simulink library "alfa_window_in"  (R2013b)
settings: Solver=ode45  StartTime=0.0  StopTime=10.0  RelTol=1e-3
settings Model: Creator=lena.frank  LastModifiedBy=drhf

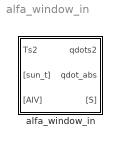
== system alfa_window_in ==
  alfa_window_in : Subsystem  mask(ALFA){gvalue=0.7, emission_in=0.87, wallsurface=1, frame=0.1, numlayer=2}
      mask prompts: gvalue "Energy transmission by sunlight (g-value) 0..1"; emission_in "Longwave emissivity (0..1)"; wallsurface "Surface of the window (with frame) in m²"; frame "Share of the frame on the surface (0...1)"; numlayer "Number of glass panes"
      mask help:
      | Convective and radiative heat transfer at the INDOOR SURFACE OF A VERTICAL WINDOW with 1-4 layers (each 3 ... 8 mm thick).
      |
      | Ts  : temperature of window surface, °C,
      | [sun_t]  : sun data (incidence angle, direct and diffuse radiation
      |     at tilted window surface),
      | [AIV]  : conditions of zone node,
      | qdots  : specific heat flow into window construction, W/m^2,
      | qdot_abs : specific irradiation absorption within window
      |     construction,  W/m^2,
      | [S]  : heat and air flow to zone node.

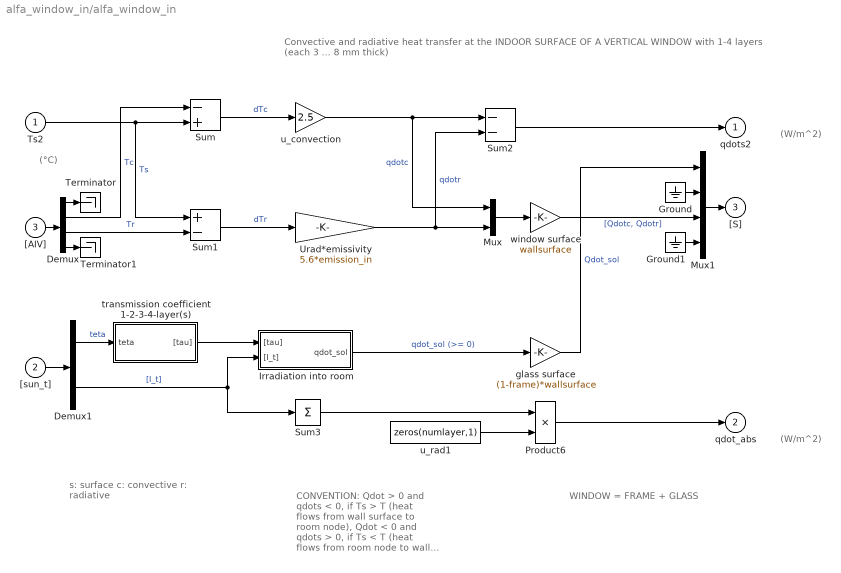
== system alfa_window_in/alfa_window_in ==
  note: (°C)
  note: Convective and radiative heat transfer at the INDOOR SURFACE OF A VERTICAL WINDOW
      | with 1-4 layers (each 3 ... 8 mm thick)
  note: (W/m^2)
  note: WINDOW = FRAME + GLASS
  note: s: surface
      | c: convective
      | r: radiative
  note: CONVENTION:
      | Qdot > 0 and qdots < 0, if Ts > T (heat flows from wall surface to room node),
      | Qdot < 0 and qdots > 0, if Ts < T (heat flows from room node to wall surface).
  note: (W/m^2)
  Ts2 : Inport
  "[sun_t]" : Inport  Port=2
  "[AIV]" : Inport  Port=3
  " glass surface" : Gain  Gain=(1-frame)*wallsurface  SaturateOnIntegerOverflow=on  OutDataTypeStr=Inherit: Same as input  ParamDataTypeStr=Inherit: Same as input
  Demux : Demux  Outputs=[1 1 1 6]
  Demux1 : Demux  Outputs=[1 2]
  Ground : Ground
  Ground1 : Ground
  Irradiation into room : Subsystem
  Mux : Mux  Inputs=2
  Mux1 : Mux  Inputs=[1 5 2 5]
  Product6 : Product  SaturateOnIntegerOverflow=on  InputSameDT=on  OutDataTypeStr=Inherit: Same as first input
  Sum : Sum  Inputs=-+  SaturateOnIntegerOverflow=on  InputSameDT=on  OutDataTypeStr=Inherit: Same as first input
  Sum1 : Sum  Inputs=+-  SaturateOnIntegerOverflow=on  InputSameDT=on  OutDataTypeStr=Inherit: Same as first input
  Sum2 : Sum  Inputs=--  SaturateOnIntegerOverflow=on  InputSameDT=on  OutDataTypeStr=Inherit: Same as first input
  Sum3 : Sum  Inputs=1  SaturateOnIntegerOverflow=on  InputSameDT=on  OutDataTypeStr=Inherit: Same as first input
  Terminator : Terminator
  Terminator1 : Terminator
  Urad*emissivity : Gain  Gain=5.6*emission_in  SaturateOnIntegerOverflow=on  OutDataTypeStr=Inherit: Same as input  ParamDataTypeStr=Inherit: Same as input
  transmission coefficient 1-2-3-4-layer(s) : Subsystem
  u_convection : Gain  Gain=2.5  SaturateOnIntegerOverflow=on  OutDataTypeStr=Inherit: Same as input  ParamDataTypeStr=Inherit: Same as input
  u_rad1 : Constant  Value=zeros(numlayer,1)
  window surface : Gain  Gain=wallsurface  SaturateOnIntegerOverflow=on  OutDataTypeStr=Inherit: Same as input  ParamDataTypeStr=Inherit: Same as input
  qdots2 : Outport
  qdot_abs : Outport  Port=2
  "[S]" : Outport  Port=3
  wires:
  transmission coefficient 1-2-3-4-layer(s)/1("[tau]") -> Irradiation into room/1("[tau]")
  Demux1/2 -> Sum3/1, Irradiation into room/2("[I_t]")  "[I_t]"
  Demux/3 -> Sum1/2  "Tr"
  Sum/1 -> u_convection/1  "dTc"
  u_rad1/1 -> Product6/2
  Demux/2 -> Sum/1  "Tc"
  window surface/1 -> Mux1/3  "[Qdotc, Qdotr]"
  " glass surface"/1 -> Mux1/1  "Qdot_sol"
  "[sun_t]"/1 -> Demux1/1
  Demux1/1 -> transmission coefficient 1-2-3-4-layer(s)/1(teta)  "teta"
  Irradiation into room/1(qdot_sol) -> " glass surface"/1  "qdot_sol (>= 0)"
  u_convection/1 -> Sum2/1, Mux/1  "qdotc"
  Urad*emissivity/1 -> Mux/2, Sum2/2  "qdotr"
  Ts2/1 -> Sum1/1, Sum/2  "Ts"
  Sum1/1 -> Urad*emissivity/1  "dTr"
  Mux/1 -> window surface/1
  Demux/1 -> Terminator/1
  "[AIV]"/1 -> Demux/1
  Demux/4 -> Terminator1/1
  Sum2/1 -> qdots2/1
  Mux1/1 -> "[S]"/1
  Ground/1 -> Mux1/2
  Ground1/1 -> Mux1/4
  Product6/1 -> qdot_abs/1
  Sum3/1 -> Product6/1

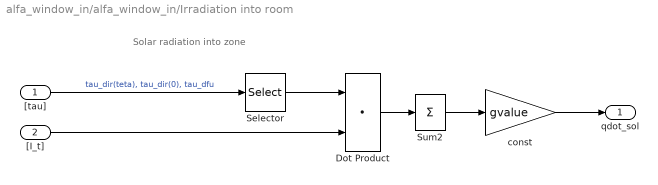
== system alfa_window_in/alfa_window_in/Irradiation into room ==
  note: Solar radiation into zone
  "[tau]" : Inport
  "[I_t]" : Inport  Port=2
  Dot Product : DotProduct  InputSameDT=on  OutDataTypeStr=Inherit: Inherit via internal rule
  Selector : Selector  InputPortWidth=3  IndexOptions=Index vector (dialog)  Indices=[1 3]  OutputSizes=1
  Sum2 : Sum  Inputs=1  SaturateOnIntegerOverflow=on  InputSameDT=on  OutDataTypeStr=Inherit: Same as first input
  const : Gain  Gain=gvalue  SaturateOnIntegerOverflow=on  OutDataTypeStr=Inherit: Same as input  ParamDataTypeStr=Inherit: Same as input
  qdot_sol : Outport
  wires:
  "[I_t]"/1 -> Dot Product/2
  "[tau]"/1 -> Selector/1  "tau_dir(teta), tau_dir(0), tau_dfu"
  Selector/1 -> Dot Product/1
  Dot Product/1 -> Sum2/1
  Sum2/1 -> const/1
  const/1 -> qdot_sol/1

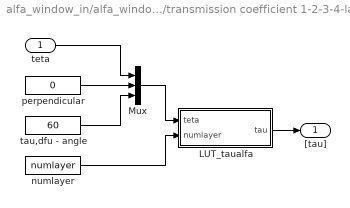
== system alfa_window_in/alfa_window_in/transmission coefficient 1-2-3-4-layer(s) ==
  teta : Inport
  LUT_taualfa : Subsystem  mask(LOOK UP TABLE){}
      mask help:
      | This block delivers the standardized LIGHT TRANSMISSION COEFFICIENT of a window glass with 1, 2, 3 or 4 layers depending on the incidence angle. Each layer may be 3 to 8 mm thick.
      |
      | teta:    incidence angle = angle between surface normal and
      |                 incidence, degree
      | numlayer: number of layers within the window glass, [1,4].
      | tau:    transmission of glass layer stack, [0,1]
  Mux : Mux  Inputs=3
  numlayer : Constant  Value=numlayer
  perpendicular : Constant  Value=0
  tau,dfu - angle : Constant  Value=60
  "[tau]" : Outport
  wires:
  teta/1 -> Mux/1
  tau,dfu - angle/1 -> Mux/3
  perpendicular/1 -> Mux/2
  Mux/1 -> LUT_taualfa/1(teta)
  numlayer/1 -> LUT_taualfa/2(numlayer)
  LUT_taualfa/1(tau) -> "[tau]"/1

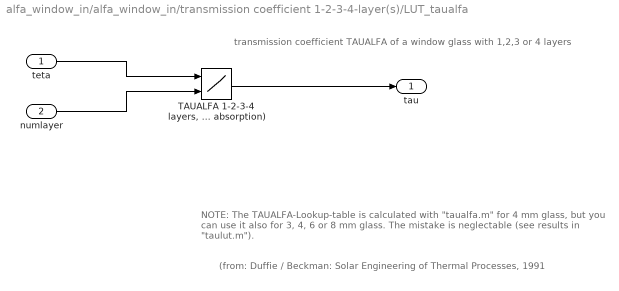
== system alfa_window_in/alfa_window_in/transmission coefficient 1-2-3-4-layer(s)/LUT_taualfa ==
  note: (from: Duffie / Beckman: Solar Engineering of Thermal Processes, 1991
  note: transmission coefficient TAUALFA of a window glass with 1,2,3 or 4 layers
  note: NOTE: The TAUALFA-Lookup-table is calculated with "taualfa.m"
      | for 4 mm glass, but you can use it also for  3, 4, 6 or 8 mm glass.
      | The mistake is neglectable (see results in "taulut.m").
  teta : Inport
  numlayer : Inport  Port=2
  "TAUALFA 1-2-3-4 layers, standardized to 1.0, (4 mm float glass, no dirt absorption, 97% room absorption)" : Lookup2D  RowIndex=[0:10:90]  ColumnIndex=[1:4]  Table=[1.0000 1.0000 1.0000 1.0000; 0.9996 0.9991 0.9987 0.9983; 0.9979 0.9961 0.9945 0.9929; 0.9937 0.9894 0.9861 0.9836; 0.9839 0.9753 0.9704 0.9680; 0.9608 0.9438 0.9365 0.9361; 0.9061 0.8679 0.8484 0.8413; 0.7755 0.6821 0.6182 0.5717; 0.4807 0.3277 0.2324 0.1688; 0 0 0 0]  SaturateOnIntegerOverflow=on  InputSameDT=on
  tau : Outport
  wires:
  "TAUALFA 1-2-3-4 layers, standardized to 1.0, (4 mm float glass, no dirt absorption, 97% room absorption)"/1 -> tau/1
  numlayer/1 -> "TAUALFA 1-2-3-4 layers, standardized to 1.0, (4 mm float glass, no dirt absorption, 97% room absorption)"/2
  teta/1 -> "TAUALFA 1-2-3-4 layers, standardized to 1.0, (4 mm float glass, no dirt absorption, 97% room absorption)"/1
